simulink model "automata_learning"  (R2022a)
(part 6 of 10)

(exp(0.5672950148582458 * x2 - 0.3294227719306946 * x1 + 0.08456141501665115) + 1.0) + 0.500249445438385 * (exp(0.6337171792984009 * x2 - 0.6585735082626343 * x1 + 0.07681625336408615) - 1.0) / (exp(0.6337171792984009 * x2 - 0.6585735082626343 * x1 + 0.07681625336408615) + 1.0) - 0.16290931403636932 * (exp(0.3557380735874176 * x1 + 0.5222645998001099 * x2 - 0.001446970272809267) - 1.0) / (exp(0.3557380735874176 * x1 + 0.5222645998001099 * x2 - 0.001446970272809267) + 1.0) + 0.038993220776319504 * (exp(0.18025468289852142 * x1 - 0.3242053985595703 * x2 + 0.15187674760818481) - 1.0) / (exp(0.18025468289852142 * x1 - 0.3242053985595703 * x2 + 0.15187674760818481) + 1.0) + 0.46942368149757385 * (exp(0.07163150608539581 * x1 - 0.003734872443601489 * x2 + 0.2506158649921417) - 1.0) / (exp(0.07163150608539581 * x1 - 0.003734872443601489 * x2 + 0.2506158649921417) + 1.0) + 0.284322589635849 * (exp(0.5243523120880127 * x1 + 0.3820697069168091 * x2 - 0.049405328929424286) - 1.0) / (exp(0.5243523120880127 * x1 + 0.3820697069168091 * x2 - 0.049405328929424286) + 1.0) - 0.21226757764816284 * (exp(0.15946464240550995 * x1 + 0.699800431728363 * x2 - 0.09449707716703415) - 1.0) / (exp(0.15946464240550995 * x1 + 0.699800431728363 * x2 - 0.09449707716703415) + 1.0) + 0.007218976970762014 * (exp(0.5389211177825928 * x1 - 0.7707962393760681 * x2 + 0.100162573158741) - 1.0) / (exp(0.5389211177825928 * x1 - 0.7707962393760681 * x2 + 0.100162573158741) + 1.0) - 0.21847893297672272 * (exp(0.46924644708633423 * x1 + 0.2838100492954254 * x2 + 0.15894784033298492) - 1.0) / (exp(0.46924644708633423 * x1 + 0.2838100492954254 * x2 + 0.15894784033298492) + 1.0) + 0.8710818886756897 * (exp(0.2737453579902649 * x1 - 0.6708545684814453 * x2 + 0.23592641949653625) - 1.0) / (exp(0.2737453579902649 * x1 - 0.6708545684814453 * x2 + 0.23592641949653625) + 1.0) + 0.9388759732246399 * (exp(0.15929313004016876 * x1 + 0.3402467966079712 * x2 + 0.21554578840732574) - 1.0) / (exp(0.15929313004016876 * x1 + 0.3402467966079712 * x2 + 0.21554578840732574) + 1.0) + 0.7285745143890381 * (exp(0.2647458612918854 * x1 + 0.06048266217112541 * x2 - 0.1825292855501175) - 1.0) / (exp(0.2647458612918854 * x1 + 0.06048266217112541 * x2 - 0.1825292855501175) + 1.0) + 0.1003083735704422 * (exp(0.14216692745685577 * x1 + 0.7861806750297546 * x2 - 0.21987329423427582) - 1.0) / (exp(0.14216692745685577 * x1 + 0.7861806750297546 * x2 - 0.21987329423427582) + 1.0) + 0.3721664845943451 * (exp(0.23872555792331696 * x2 - 0.15653954446315765 * x1 + 0.18696969747543335) - 1.0) / (exp(0.23872555792331696 * x2 - 0.15653954446315765 * x1 + 0.18696969747543335) + 1.0) + 0.4506336450576782 * (exp(0.028650518506765366 * x2 - 0.221619114279747 * x1 + 0.14330333471298218) - 1.0) / (exp(0.028650518506765366 * x2 - 0.221619114279747 * x1 + 0.14330333471298218) + 1.0) - 0.38137251138687134 * (exp(0.45747116208076477 * x2 - 0.594399094581604 * x1 + 0.23476329445838928) - 1.0) / (exp(0.45747116208076477 * x2 - 0.594399094581604 * x1 + 0.23476329445838928) + 1.0) - 0.5165428519248962 * (exp(0.46693146228790283 * x1 + 0.358431339263916 * x2 + 0.4691663682460785) - 1.0) / (exp(0.46693146228790283 * x1 + 0.358431339263916 * x2 + 0.4691663682460785) + 1.0) + 0.08895933628082275) + 1.0) - 0.38439175486564636 * (exp(0.9460711479187012 * (exp(0.032108455896377563 * x2 - 0.07343825697898865 * x1 + 0.15331247448921204) - 1.0) / (exp(0.032108455896377563 * x2 - 0.07343825697898865 * x1 + 0.15331247448921204) + 1.0) + 0.7185744047164917 * (exp(0.1574449986219406 * x2 - 0.5194829702377319 * x1 + 0.14603400230407715) - 1.0) / (exp(0.1574449986219406 * x2 - 0.5194829702377319 * x1 + 0.14603400230407715) + 1.0) - 0.5400316119194031 * (exp(0.38573387265205383 * x1 - 0.14479495584964752 * x2 + 0.12680158019065857) - 1.0) / (exp(0.38573387265205383 * x1 - 0.14479495584964752 * x2 + 0.12680158019065857) + 1.0) + 0.43772217631340027 * (exp(0.5672950148582458 * x2 - 0.3294227719306946 * x1 + 0.08456141501665115) - 1.0) / (exp(0.5672950148582458 * x2 - 0.3294227719306946 * x1 + 0.08456141501665115) + 1.0) + 0.005960926879197359 * (exp(0.6337171792984009 * x2 - 0.6585735082626343 * x1 + 0.07681625336408615) - 1.0) / (exp(0.6337171792984009 * x2 - 0.6585735082626343 * x1 + 0.07681625336408615) + 1.0) + 0.40139031410217285 * (exp(0.3557380735874176 * x1 + 0.5222645998001099 * x2 - 0.001446970272809267) - 1.0) / (exp(0.3557380735874176 * x1 + 0.5222645998001099 * x2 - 0.001446970272809267) + 1.0) + 0.5896893739700317 * (exp(0.18025468289852142 * x1 - 0.3242053985595703 * x2 + 0.15187674760818481) - 1.0) / (exp(0.18025468289852142 * x1 - 0.3242053985595703 * x2 + 0.15187674760818481) + 1.0) + 0.41773173213005066 * (exp(0.07163150608539581 * x1 - 0.003734872443601489 * x2 + 0.2506158649921417) - 1.0) / (exp(0.07163150608539581 * x1 - 0.003734872443601489 * x2 + 0.2506158649921417) + 1.0) - 0.28515946865081787 * (exp(0.5243523120880127 * x1 + 0.3820697069168091 * x2 - 0.049405328929424286) - 1.0) / (exp(0.5243523120880127 * x1 + 0.3820697069168091 * x2 - 0.049405328929424286) + 1.0) + 0.2827272117137909 * (exp(0.15946464240550995 * x1 + 0.699800431728363 * x2 - 0.09449707716703415) - 1.0) / (exp(0.15946464240550995 * x1 + 0.699800431728363 * x2 - 0.09449707716703415) + 1.0) + 0.08473894745111465 * (exp(0.5389211177825928 * x1 - 0.7707962393760681 * x2 + 0.100162573158741) - 1.0) / (exp(0.5389211177825928 * x1 - 0.7707962393760681 * x2 + 0.100162573158741) + 1.0) - 0.12469436973333359 * (exp(0.46924644708633423 * x1 + 0.2838100492954254 * x2 + 0.15894784033298492) - 1.0) / (exp(0.46924644708633423 * x1 + 0.2838100492954254 * x2 + 0.15894784033298492) + 1.0) + 0.4589995741844177 * (exp(0.2737453579902649 * x1 - 0.6708545684814453 * x2 + 0.23592641949653625) - 1.0) / (exp(0.2737453579902649 * x1 - 0.6708545684814453 * x2 + 0.23592641949653625) + 1.0) - 0.09170734882354736 * (exp(0.15929313004016876 * x1 + 0.3402467966079712 * x2 + 0.21554578840732574) - 1.0) / (exp(0.15929313004016876 * x1 + 0.3402467966079712 * x2 + 0.21554578840732574) + 1.0) - 0.8364236354827881 * (exp(0.2647458612918854 * x1 + 0.06048266217112541 * x2 - 0.1825292855501175) - 1.0) / (exp(0.2647458612918854 * x1 + 0.06048266217112541 * x2 - 0.1825292855501175) + 1.0) - 0.7059954404830933 * (exp(0.14216692745685577 * x1 + 0.7861806750297546 * x2 - 0.21987329423427582) - 1.0) / (exp(0.14216692745685577 * x1 + 0.7861806750297546 * x2 - 0.21987329423427582) + 1.0) - 0.234619140625 * (exp(0.23872555792331696 * x2 - 0.15653954446315765 * x1 + 0.18696969747543335) - 1.0) / (exp(0.23872555792331696 * x2 - 0.15653954446315765 * x1 + 0.18696969747543335) + 1.0) + 0.47808125615119934 * (exp(0.028650518506765366 * x2 - 0.221619114279747 * x1 + 0.14330333471298218) - 1.0) / (exp(0.028650518506765366 * x2 - 0.221619114279747 * x1 + 0.14330333471298218) + 1.0) + 0.6417360305786133 * (exp(0.45747116208076477 * x2 - 0.594399094581604 * x1 + 0.23476329445838928) - 1.0) / (exp(0.45747116208076477 * x2 - 0.594399094581604 * x1 + 0.23476329445838928) + 1.0) + 0.3669280707836151 * (exp(0.46693146228790283 * x1 + 0.358431339263916 * x2 + 0.4691663682460785) - 1.0) / (exp(0.46693146228790283 * x1 + 0.358431339263916 * x2 + 0.4691663682460785) + 1.0) + 0.14854967594146729) - 1.0) / (exp(0.9460711479187012 * (exp(0.032108455896377563 * x2 - 0.07343825697898865 * x1 + 0.15331247448921204) - 1.0) / (exp(0.032108455896377563 * x2 - 0.07343825697898865 * x1 + 0.15331247448921204) + 1.0) + 0.7185744047164917 * (exp(0.1574449986219406 * x2 - 0.5194829702377319 * x1 + 0.14603400230407715) - 1.0) / (exp(0.1574449986219406 * x2 - 0.5194829702377319 * x1 + 0.14603400230407715) + 1.0) - 0.5400316119194031 * (exp(0.38573387265205383 * x1 - 0.14479495584964752 * x2 + 0.12680158019065857) - 1.0) / (exp(0.38573387265205383 * x1 - 0.14479495584964752 * x2 + 0.12680158019065857) + 1.0) + 0.43772217631340027 * (exp(0.5672950148582458 * x2 - 0.3294227719306946 * x1 + 0.08456141501665115) - 1.0) / (exp(0.5672950148582458 * x2 - 0.3294227719306946 * x1 + 0.08456141501665115) + 1.0) + 0.005960926879197359 * (exp(0.6337171792984009 * x2 - 0.6585735082626343 * x1 + 0.07681625336408615) - 1.0) / (exp(0.6337171792984009 * x2 - 0.6585735082626343 * x1 + 0.07681625336408615) + 1.0) + 0.40139031410217285 * (exp(0.3557380735874176 * x1 + 0.5222645998001099 * x2 - 0.001446970272809267) - 1.0) / (exp(0.3557380735874176 * x1 + 0.5222645998001099 * x2 - 0.001446970272809267) + 1.0) + 0.5896893739700317 * (exp(0.18025468289852142 * x1 - 0.3242053985595703 * x2 + 0.15187674760818481) - 1.0) / (exp(0.18025468289852142 * x1 - 0.3242053985595703 * x2 + 0.15187674760818481) + 1.0) + 0.41773173213005066 * (exp(0.07163150608539581 * x1 - 0.003734872443601489 * x2 + 0.2506158649921417) - 1.0) / (exp(0.07163150608539581 * x1 - 0.003734872443601489 * x2 + 0.2506158649921417) + 1.0) - 0.28515946865081787 * (exp(0.5243523120880127 * x1 + 0.3820697069168091 * x2 - 0.049405328929424286) - 1.0) / (exp(0.5243523120880127 * x1 + 0.3820697069168091 * x2 - 0.049405328929424286) + 1.0) + 0.2827272117137909 * (exp(0.15946464240550995 * x1 + 0.699800431728363 * x2 - 0.09449707716703415) - 1.0) / (exp(0.15946464240550995 * x1 + 0.699800431728363 * x2 - 0.09449707716703415) + 1.0) + 0.08473894745111465 * (exp(0.5389211177825928 * x1 - 0.7707962393760681 * x2 + 0.100162573158741) - 1.0) / (exp(0.5389211177825928 * x1 - 0.7707962393760681 * x2 + 0.100162573158741) + 1.0) - 0.12469436973333359 * (exp(0.46924644708633423 * x1 + 0.2838100492954254 * x2 + 0.15894784033298492) - 1.0) / (exp(0.46924644708633423 * x1 + 0.2838100492954254 * x2 + 0.15894784033298492) + 1.0) + 0.4589995741844177 * (exp(0.2737453579902649 * x1 - 0.6708545684814453 * x2 + 0.23592641949653625) - 1.0) / (exp(0.2737453579902649 * x1 - 0.6708545684814453 * x2 + 0.23592641949653625) + 1.0) - 0.09170734882354736 * (exp(0.15929313004016876 * x1 + 0.3402467966079712 * x2 + 0.21554578840732574) - 1.0) / (exp(0.15929313004016876 * x1 + 0.3402467966079712 * x2 + 0.21554578840732574) + 1.0) - 0.8364236354827881 * (exp(0.2647458612918854 * x1 + 0.06048266217112541 * x2 - 0.1825292855501175) - 1.0) / (exp(0.2647458612918854 * x1 + 0.06048266217112541 * x2 - 0.1825292855501175) + 1.0) - 0.7059954404830933 * (exp(0.14216692745685577 * x1 + 0.7861806750297546 * x2 - 0.21987329423427582) - 1.0) / (exp(0.14216692745685577 * x1 + 0.7861806750297546 * x2 - 0.21987329423427582) + 1.0) - 0.234619140625 * (exp(0.23872555792331696 * x2 - 0.15653954446315765 * x1 + 0.18696969747543335) - 1.0) / (exp(0.23872555792331696 * x2 - 0.15653954446315765 * x1 + 0.18696969747543335) + 1.0) + 0.47808125615119934 * (exp(0.028650518506765366 * x2 - 0.221619114279747 * x1 + 0.14330333471298218) - 1.0) / (exp(0.028650518506765366 * x2 - 0.221619114279747 * x1 + 0.14330333471298218) + 1.0) + 0.6417360305786133 * (exp(0.45747116208076477 * x2 - 0.594399094581604 * x1 + 0.23476329445838928) - 1.0) / (exp(0.45747116208076477 * x2 - 0.594399094581604 * x1 + 0.23476329445838928) + 1.0) + 0.3669280707836151 * (exp(0.46693146228790283 * x1 + 0.358431339263916 * x2 + 0.4691663682460785) - 1.0) / (exp(0.46693146228790283 * x1 + 0.358431339263916 * x2 + 0.4691663682460785) + 1.0) + 0.14854967594146729) + 1.0) + 0.3899663984775543 * (exp(0.13915207982063293 * (exp(0.032108455896377563 * x2 - 0.07343825697898865 * x1 + 0.15331247448921204) - 1.0) / (exp(0.032108455896377563 * x2 - 0.07343825697898865 * x1 + 0.15331247448921204) + 1.0) - 0.013549529947340488 * (exp(0.1574449986219406 * x2 - 0.5194829702377319 * x1 + 0.14603400230407715) - 1.0) / (exp(0.1574449986219406 * x2 - 0.5194829702377319 * x1 + 0.14603400230407715) + 1.0) + 0.45576003193855286 * (exp(0.38573387265205383 * x1 - 0.14479495584964752 * x2 + 0.12680158019065857) - 1.0) / (exp(0.38573387265205383 * x1 - 0.14479495584964752 * x2 + 0.12680158019065857) + 1.0) + 0.5031511783599854 * (exp(0.5672950148582458 * x2 - 0.3294227719306946 * x1 + 0.08456141501665115) - 1.0) / (exp(0.5672950148582458 * x2 - 0.3294227719306946 * x1 + 0.08456141501665115) + 1.0) - 0.19170700013637543 * (exp(0.6337171792984009 * x2 - 0.6585735082626343 * x1 + 0.07681625336408615) - 1.0) / (exp(0.6337171792984009 * x2 - 0.6585735082626343 * x1 + 0.07681625336408615) + 1.0) + 0.2848758101463318 * (exp(0.3557380735874176 * x1 + 0.5222645998001099 * x2 - 0.001446970272809267) - 1.0) / (exp(0.3557380735874176 * x1 + 0.5222645998001099 * x2 - 0.001446970272809267) + 1.0) - 0.5725408792495728 * (exp(0.18025468289852142 * x1 - 0.3242053985595703 * x2 + 0.15187674760818481) - 1.0) / (exp(0.18025468289852142 * x1 - 0.3242053985595703 * x2 + 0.15187674760818481) + 1.0) + 0.6819994449615479 * (exp(0.07163150608539581 * x1 - 0.003734872443601489 * x2 + 0.2506158649921417) - 1.0) / (exp(0.07163150608539581 * x1 - 0.003734872443601489 * x2 + 0.2506158649921417) + 1.0) + 0.48650869727134705 * (exp(0.5243523120880127 * x1 + 0.3820697069168091 * x2 - 0.049405328929424286) - 1.0) / (exp(0.5243523120880127 * x1 + 0.3820697069168091 * x2 - 0.049405328929424286) + 1.0) - 0.49587011337280273 * (exp(0.15946464240550995 * x1 + 0.699800431728363 * x2 - 0.09449707716703415) - 1.0) / (exp(0.15946464240550995 * x1 + 0.699800431728363 * x2 - 0.09449707716703415) + 1.0) + 0.32867637276649475 * (exp(0.5389211177825928 * x1 - 0.7707962393760681 * x2 + 0.100162573158741) - 1.0) / (exp(0.5389211177825928 * x1 - 0.7707962393760681 * x2 + 0.100162573158741) + 1.0) + 0.12904153764247894 * (exp(0.46924644708633423 * x1 + 0.2838100492954254 * x2 + 0.15894784033298492) - 1.0) / (exp(0.46924644708633423 * x1 + 0.2838100492954254 * x2 + 0.15894784033298492) + 1.0) - 0.4668161869049072 * (exp(0.2737453579902649 * x1 - 0.6708545684814453 * x2 + 0.23592641949653625) - 1.0) / (exp(0.2737453579902649 * x1 - 0.6708545684814453 * x2 + 0.23592641949653625) + 1.0) + 0.8701659440994263 * (exp(0.15929313004016876 * x1 + 0.3402467966079712 * x2 + 0.21554578840732574) - 1.0) / (exp(0.15929313004016876 * x1 + 0.3402467966079712 * x2 + 0.21554578840732574) + 1.0) + 1.0214658975601196 * (exp(0.2647458612918854 * x1 + 0.06048266217112541 * x2 - 0.1825292855501175) - 1.0) / (exp(0.2647458612918854 * x1 + 0.06048266217112541 * x2 - 0.1825292855501175) + 1.0) + 0.3350728154182434 * (exp(0.14216692745685577 * x1 + 0.7861806750297546 * x2 - 0.21987329423427582) - 1.0) / (exp(0.14216692745685577 * x1 + 0.7861806750297546 * x2 - 0.21987329423427582) + 1.0) - 0.5930564999580383 * (exp(0.23872555792331696 * x2 - 0.15653954446315765 * x1 + 0.18696969747543335) - 1.0) / (exp(0.23872555792331696 * x2 - 0.15653954446315765 * x1 + 0.18696969747543335) + 1.0) + 0.0021656707394868135 * (exp(0.028650518506765366 * x2 - 0.221619114279747 * x1 + 0.14330333471298218) - 1.0) / (exp(0.028650518506765366 * x2 - 0.221619114279747 * x1 + 0.14330333471298218) + 1.0) + 0.5999830365180969 * (exp(0.45747116208076477 * x2 - 0.594399094581604 * x1 + 0.23476329445838928) - 1.0) / (exp(0.45747116208076477 * x2 - 0.594399094581604 * x1 + 0.23476329445838928) + 1.0) - 0.2212107628583908 * (exp(0.46693146228790283 * x1 + 0.358431339263916 * x2 + 0.4691663682460785) - 1.0) / (exp(0.46693146228790283 * x1 + 0.358431339263916 * x2 + 0.4691663682460785) + 1.0) + 0.0015353158814832568) - 1.0) / (exp(0.13915207982063293 * (exp(0.032108455896377563 * x2 - 0.07343825697898865 * x1 + 0.15331247448921204) - 1.0) / (exp(0.032108455896377563 * x2 - 0.07343825697898865 * x1 + 0.15331247448921204) + 1.0) - 0.013549529947340488 * (exp(0.1574449986219406 * x2 - 0.5194829702377319 * x1 + 0.14603400230407715) - 1.0) / (exp(0.1574449986219406 * x2 - 0.5194829702377319 * x1 + 0.14603400230407715) + 1.0) + 0.45576003193855286 * (exp(0.38573387265205383 * x1 - 0.14479495584964752 * x2 + 0.12680158019065857) - 1.0) / (exp(0.38573387265205383 * x1 - 0.14479495584964752 * x2 + 0.12680158019065857) + 1.0) + 0.5031511783599854 * (exp(0.5672950148582458 * x2 - 0.3294227719306946 * x1 + 0.08456141501665115) - 1.0) / (exp(0.5672950148582458 * x2 - 0.3294227719306946 * x1 + 0.08456141501665115) + 1.0) - 0.19170700013637543 * (exp(0.6337171792984009 * x2 - 0.6585735082626343 * x1 + 0.07681625336408615) - 1.0) / (exp(0.6337171792984009 * x2 - 0.6585735082626343 * x1 + 0.07681625336408615) + 1.0) + 0.2848758101463318 * (exp(0.3557380735874176 * x1 + 0.5222645998001099 * x2 - 0.001446970272809267) - 1.0) / (exp(0.3557380735874176 * x1 + 0.5222645998001099 * x2 - 0.001446970272809267) + 1.0) - 0.5725408792495728 * (exp(0.18025468289852142 * x1 - 0.3242053985595703 * x2 + 0.15187674760818481) - 1.0) / (exp(0.18025468289852142 * x1 - 0.3242053985595703 * x2 + 0.15187674760818481) + 1.0) + 0.6819994449615479 * (exp(0.07163150608539581 * x1 - 0.003734872443601489 * x2 + 0.2506158649921417) - 1.0) / (exp(0.07163150608539581 * x1 - 0.003734872443601489 * x2 + 0.2506158649921417) + 1.0) + 0.48650869727134705 * (exp(0.5243523120880127 * x1 + 0.3820697069168091 * x2 - 0.049405328929424286) - 1.0) / (exp(0.5243523120880127 * x1 + 0.3820697069168091 * x2 - 0.049405328929424286) + 1.0) - 0.49587011337280273 * (exp(0.15946464240550995 * x1 + 0.699800431728363 * x2 - 0.09449707716703415) - 1.0) / (exp(0.15946464240550995 * x1 + 0.699800431728363 * x2 - 0.09449707716703415) + 1.0) + 0.32867637276649475 * (exp(0.5389211177825928 * x1 - 0.7707962393760681 * x2 + 0.100162573158741) - 1.0) / (exp(0.5389211177825928 * x1 - 0.7707962393760681 * x2 + 0.100162573158741) + 1.0) + 0.12904153764247894 * (exp(0.46924644708633423 * x1 + 0.2838100492954254 * x2 + 0.15894784033298492) - 1.0) / (exp(0.46924644708633423 * x1 + 0.2838100492954254 * x2 + 0.15894784033298492) + 1.0) - 0.4668161869049072 * (exp(0.2737453579902649 * x1 - 0.6708545684814453 * x2 + 0.23592641949653625) - 1.0) / (exp(0.2737453579902649 * x1 - 0.6708545684814453 * x2 + 0.23592641949653625) + 1.0) + 0.8701659440994263 * (exp(0.15929313004016876 * x1 + 0.3402467966079712 * x2 + 0.21554578840732574) - 1.0) / (exp(0.15929313004016876 * x1 + 0.3402467966079712 * x2 + 0.21554578840732574) + 1.0) + 1.0214658975601196 * (exp(0.2647458612918854 * x1 + 0.06048266217112541 * x2 - 0.1825292855501175) - 1.0) / (exp(0.2647458612918854 * x1 + 0.06048266217112541 * x2 - 0.1825292855501175) + 1.0) + 0.3350728154182434 * (exp(0.14216692745685577 * x1 + 0.7861806750297546 * x2 - 0.21987329423427582) - 1.0) / (exp(0.14216692745685577 * x1 + 0.7861806750297546 * x2 - 0.21987329423427582) + 1.0) - 0.5930564999580383 * (exp(0.23872555792331696 * x2 - 0.15653954446315765 * x1 + 0.18696969747543335) - 1.0) / (exp(0.23872555792331696 * x2 - 0.15653954446315765 * x1 + 0.18696969747543335) + 1.0) + 0.0021656707394868135 * (exp(0.028650518506765366 * x2 - 0.221619114279747 * x1 + 0.14330333471298218) - 1.0) / (exp(0.028650518506765366 * x2 - 0.221619114279747 * x1 + 0.14330333471298218) + 1.0) + 0.5999830365180969 * (exp(0.45747116208076477 * x2 - 0.594399094581604 * x1 + 0.23476329445838928) - 1.0) / (exp(0.45747116208076477 * x2 - 0.594399094581604 * x1 + 0.23476329445838928) + 1.0) - 0.2212107628583908 * (exp(0.46693146228790283 * x1 + 0.358431339263916 * x2 + 0.4691663682460785) - 1.0) / (exp(0.46693146228790283 * x1 + 0.358431339263916 * x2 + 0.4691663682460785) + 1.0) + 0.0015353158814832568) + 1.0) + 0.05681779235601425;
    x1_out=x1;
    x2_out=x2;
    automata_learning_location =1;
  state loc2
    du:
